simulink library "simulink_control_blocks_lib"  (R2025a)
settings: Solver=VariableStepAuto  StartTime=0.0  StopTime=10.0  RelTol=1e-3
settings Model: Creator=xing2  LastModifiedBy=xing2

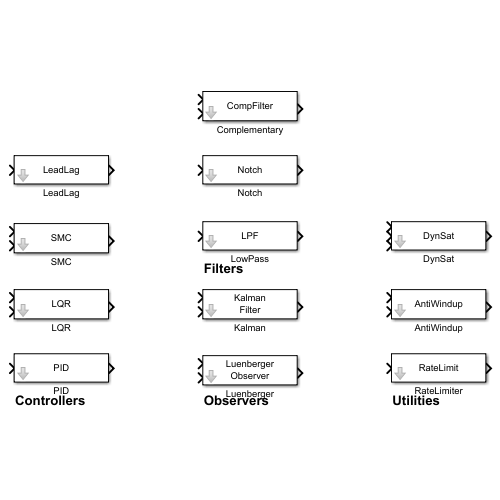
[thumbnail: Simulink's stored preview of the top-level diagram]
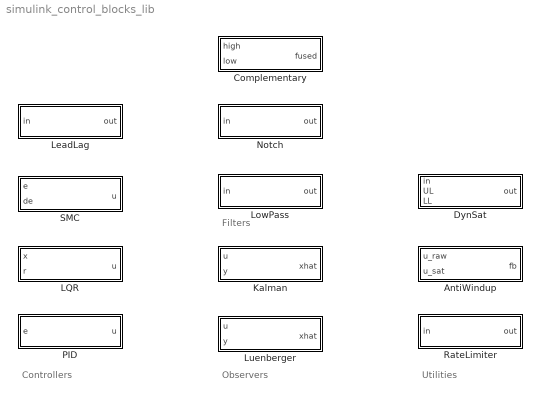
== system simulink_control_blocks_lib ==
  note: Controllers
  note: Observers
  note: Filters
  note: Utilities
  AntiWindup : Subsystem  mask{Kaw=1}
      mask help: Anti-Windup: Kaw*(u_sat-u_raw)
      mask Display: disp('AntiWindup');
  Complementary : Subsystem  mask{alpha=0.98}
      mask prompts: alpha "alpha (0~1)"
      mask help: Complementary Filter: alpha*high + (1-alpha)*low
      mask Display: disp('CompFilter');
  DynSat : Subsystem
      mask help: Dynamic Saturation with variable limits via input ports
      mask Display: disp('DynSat');
  Kalman : Subsystem  mask{A_kf=[0 1;-10 -0.5], B_aug=[0 3;1 5], C_kf=[1 0;0 1], D_aug=[0 0;0 0], x0=[0;0]}
      mask prompts: A_kf "A matrix"; B_aug "B_aug=[B K]"; C_kf "C matrix"; D_aug "D matrix"
      mask help: Kalman Filter. B_aug=[B, K_kalman] for input [u; y]
      mask Display: disp('Kalman\nFilter');
  LQR : Subsystem  mask{K_vec=[3 1], Ki=0, UL=10, LL=-10}
      mask prompts: K_vec "K vector"; Ki "Ki (integral)"; UL "Upper Limit"; LL "Lower Limit"
      mask help: LQR State Feedback Controller with integral action
      mask Display: disp('LQR');
  LeadLag : Subsystem  mask{K=1, T=0.1, alpha=3}
      mask prompts: K "Gain K"; T "Time const T"; alpha "alpha (>1=Lead)"
      mask help: Lead-Lag Compensator: Lead(alpha>1), Lag(alpha<1)
      mask Display: disp('LeadLag');
  LowPass : Subsystem  mask{wc=628}
      mask prompts: wc "Cutoff wc (rad/s)"
      mask help: 2nd-order Butterworth Low-Pass Filter
      mask Display: disp('LPF');
  Luenberger : Subsystem  mask{A_obs=[0 1;-10 -0.5], B_aug=[0 5;1 10], C_obs=[1 0;0 1], D_aug=[0 0;0 0], x0=[0;0]}
      mask prompts: A_obs "A matrix"; B_aug "B_aug=[B L]"; C_obs "C matrix"; D_aug "D matrix"
      mask help: Luenberger Observer: dxhat=A*xhat+[B,L]*[u;y]. B_aug=[B, L]
      mask Display: disp('Luenberger\nObserver');
  Notch : Subsystem  mask{wn=628, zeta1=0.01, zeta2=0.5}
      mask prompts: wn "wn (rad/s)"; zeta1 "zeta1 (notch depth)"; zeta2 "zeta2 (notch width)"
      mask help: Notch Filter: attenuate a specific frequency
      mask Display: disp('Notch');
  PID : Subsystem  mask{Kp=3, Ki=0.5, Kd=0.2, N=100, UL=10, LL=-10, Kaw=1}
      mask prompts: UL "Upper Limit"; LL "Lower Limit"; Kaw "Anti-Windup Gain"
      mask help: PID Controller with anti-windup and derivative filtering
      mask Display: disp('PID');
  RateLimiter : Subsystem  mask{R_up=1, R_down=-1}
      mask prompts: R_up "Rise rate (+)"; R_down "Fall rate (-)"
      mask help: Rate Limiter: limits signal rate via derivative+saturation+integrator
      mask Display: disp('RateLimit');
  SMC : Subsystem  mask{lambda=10, K_smc=3, phi=0.1}
      mask prompts: lambda "lambda (slope)"; K_smc "K (gain)"; phi "phi (boundary)"
      mask help: Sliding Mode Controller with boundary layer
      mask Display: disp('SMC');

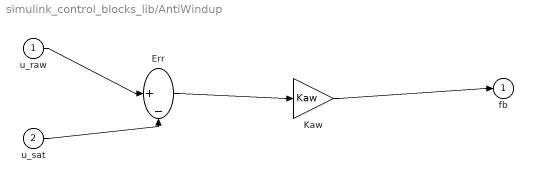
== system simulink_control_blocks_lib/AntiWindup ==
  u_raw : Inport
  u_sat : Inport  Port=2
  Err : Sum  Inputs=|+-
  Kaw : Gain  Gain=Kaw
  fb : Outport
  wires:
  Kaw/1 -> fb/1
  Err/1 -> Kaw/1
  u_sat/1 -> Err/2
  u_raw/1 -> Err/1

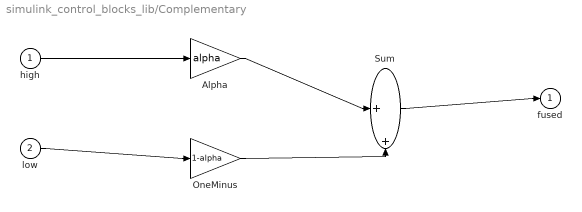
== system simulink_control_blocks_lib/Complementary ==
  high : Inport
  low : Inport  Port=2
  Alpha : Gain  Gain=alpha
  OneMinus : Gain  Gain=1-alpha
  Sum : Sum  Inputs=|++
  fused : Outport
  wires:
  Sum/1 -> fused/1
  OneMinus/1 -> Sum/2
  Alpha/1 -> Sum/1
  low/1 -> OneMinus/1
  high/1 -> Alpha/1

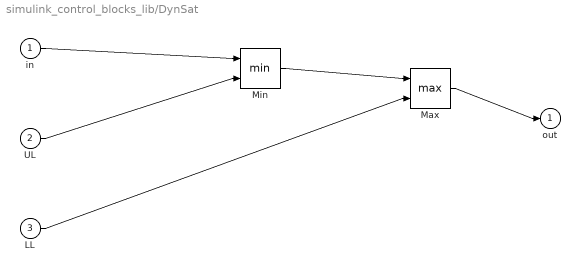
== system simulink_control_blocks_lib/DynSat ==
  in : Inport
  UL : Inport  Port=2
  LL : Inport  Port=3
  Max : MinMax  Function=max  Inputs=2
  Min : MinMax  Inputs=2
  out : Outport
  wires:
  Max/1 -> out/1
  LL/1 -> Max/2
  Min/1 -> Max/1
  UL/1 -> Min/2
  in/1 -> Min/1

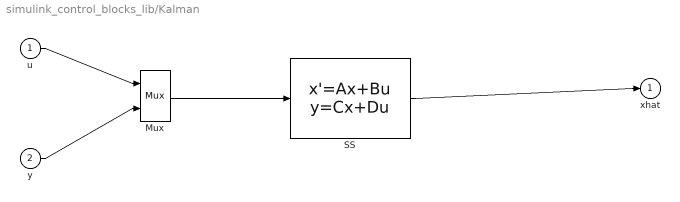
== system simulink_control_blocks_lib/Kalman ==
  u : Inport
  y : Inport  Port=2
  Mux : Mux  Inputs=2
  SS : StateSpace  A=A_kf  B=B_aug  C=C_kf  D=D_aug  InitialCondition=x0
  xhat : Outport
  wires:
  SS/1 -> xhat/1
  Mux/1 -> SS/1
  y/1 -> Mux/2
  u/1 -> Mux/1

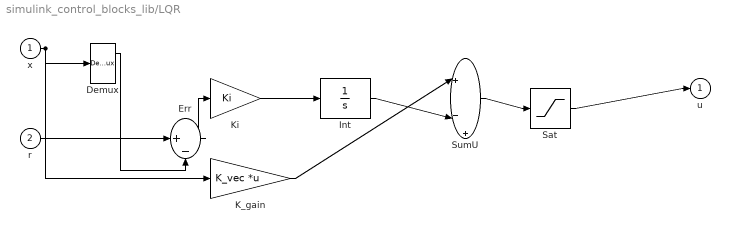
== system simulink_control_blocks_lib/LQR ==
  x : Inport
  r : Inport  Port=2
  Demux : Demux  Outputs=2
  Err : Sum  Inputs=|+-
  Int : Integrator
  K_gain : Gain  Gain=K_vec  Multiplication=Matrix(K*u)
  Ki : Gain  Gain=Ki
  Sat : Saturate  UpperLimit=UL  LowerLimit=LL
  SumU : Sum  Inputs=|+-+
  u : Outport
  wires:
  Sat/1 -> u/1
  SumU/1 -> Sat/1
  Int/1 -> SumU/2
  K_gain/1 -> SumU/1
  Ki/1 -> Int/1
  Err/1 -> Ki/1
  Demux/1 -> Err/2
  r/1 -> Err/1
  x/1 -> K_gain/1, Demux/1

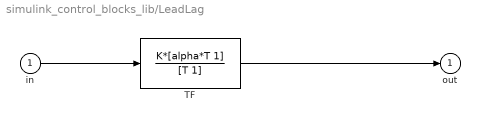
== system simulink_control_blocks_lib/LeadLag ==
  in : Inport
  TF : TransferFcn  Numerator=K*[alpha*T 1]  Denominator=[T 1]
  out : Outport
  wires:
  TF/1 -> out/1
  in/1 -> TF/1

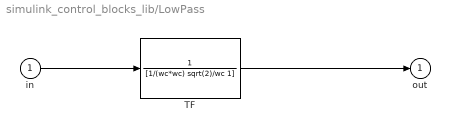
== system simulink_control_blocks_lib/LowPass ==
  in : Inport
  TF : TransferFcn  Denominator=[1/(wc*wc) sqrt(2)/wc 1]
  out : Outport
  wires:
  TF/1 -> out/1
  in/1 -> TF/1

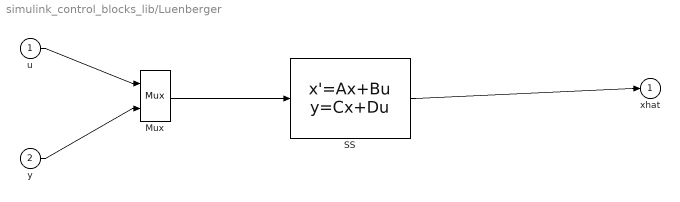
== system simulink_control_blocks_lib/Luenberger ==
  u : Inport
  y : Inport  Port=2
  Mux : Mux  Inputs=2
  SS : StateSpace  A=A_obs  B=B_aug  C=C_obs  D=D_aug  InitialCondition=x0
  xhat : Outport
  wires:
  SS/1 -> xhat/1
  Mux/1 -> SS/1
  y/1 -> Mux/2
  u/1 -> Mux/1

== system simulink_control_blocks_lib/Notch ==
  in : Inport
  TF : TransferFcn  Numerator=[1/(wn*wn) 2*zeta1/wn 1]  Denominator=[1/(wn*wn) 2*zeta2/wn 1]
  out : Outport
  wires:
  TF/1 -> out/1
  in/1 -> TF/1

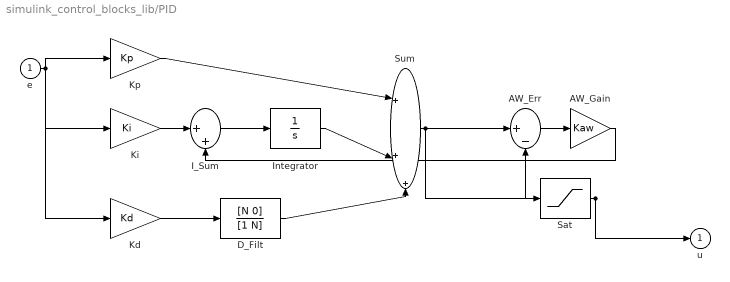
== system simulink_control_blocks_lib/PID ==
  e : Inport
  AW_Err : Sum  Inputs=|+-
  AW_Gain : Gain  Gain=Kaw
  D_Filt : TransferFcn  Numerator=[N 0]  Denominator=[1 N]
  I_Sum : Sum  Inputs=|++
  Integrator : Integrator
  Kd : Gain  Gain=Kd
  Ki : Gain  Gain=Ki
  Kp : Gain  Gain=Kp
  Sat : Saturate  UpperLimit=UL  LowerLimit=LL
  Sum : Sum  Inputs=|+++
  u : Outport
  wires:
  AW_Gain/1 -> I_Sum/2
  AW_Err/1 -> AW_Gain/1
  Sat/1 -> AW_Err/2, u/1
  Sum/1 -> AW_Err/1, Sat/1
  D_Filt/1 -> Sum/3
  Integrator/1 -> Sum/2
  Kp/1 -> Sum/1
  Kd/1 -> D_Filt/1
  I_Sum/1 -> Integrator/1
  Ki/1 -> I_Sum/1
  e/1 -> Kd/1, Ki/1, Kp/1

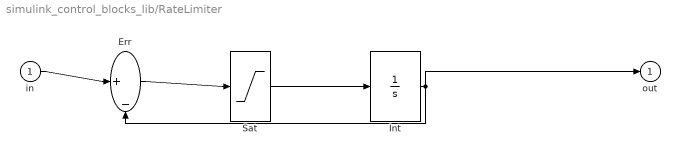
== system simulink_control_blocks_lib/RateLimiter ==
  in : Inport
  Err : Sum  Inputs=|+-
  Int : Integrator
  Sat : Saturate  UpperLimit=R_up  LowerLimit=R_down
  out : Outport
  wires:
  Int/1 -> Err/2, out/1
  Sat/1 -> Int/1
  Err/1 -> Sat/1
  in/1 -> Err/1

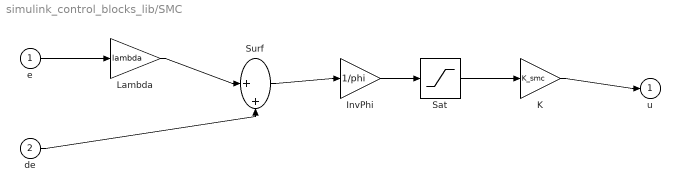
== system simulink_control_blocks_lib/SMC ==
  e : Inport
  de : Inport  Port=2
  InvPhi : Gain  Gain=1/phi
  K : Gain  Gain=K_smc
  Lambda : Gain  Gain=lambda
  Sat : Saturate  UpperLimit=1  LowerLimit=-1
  Surf : Sum  Inputs=|++
  u : Outport
  wires:
  K/1 -> u/1
  Sat/1 -> K/1
  InvPhi/1 -> Sat/1
  Surf/1 -> InvPhi/1
  de/1 -> Surf/2
  Lambda/1 -> Surf/1
  e/1 -> Lambda/1
